simulink model "untitled"  (R2023a)
settings: Solver=VariableStepAuto  StartTime=0.0  StopTime=5.0  RelTol=1e-3
libraries: dspvision x3, dspadpt3 x2, commchan3 x1
settings Model: Creator=Admin  LastModifiedBy=Admin

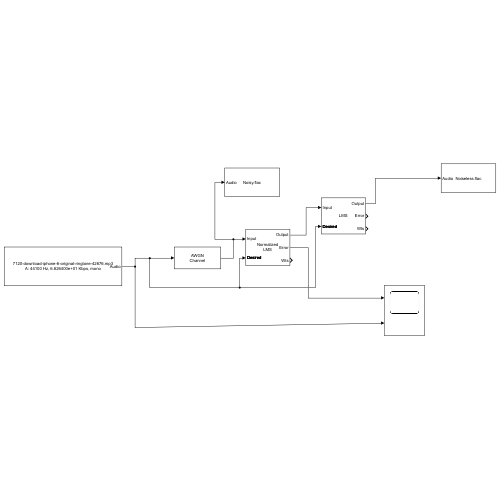
[thumbnail: Simulink's stored preview of the top-level diagram]
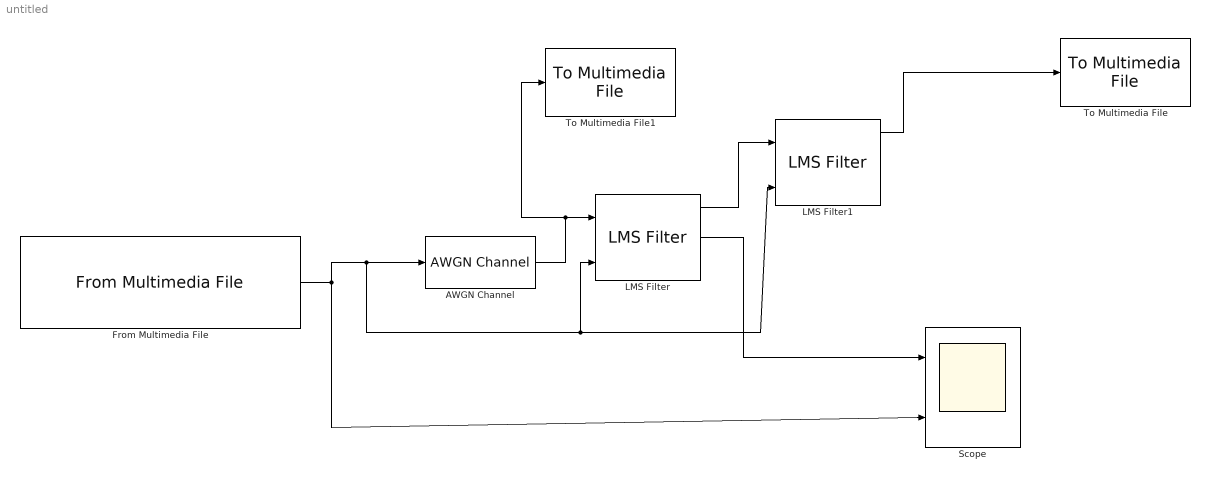
== system untitled ==
  AWGN Channel : commchan3/AWGN Channel  LegacyMode=off  NoiseMethod="Signal to noise ratio  (SNR)"  noiseMode="Signal to noise ratio  (SNR)"  EbNo=10  EsNo=10  SNR=25  BitsPerSymbol=1  SignalPower=1  SamplesPerSymbol=1  SymbolPeriod=1  VarianceSource=Parameter  Variance=1  RandomStream=Global stream  Seed=67  SimulateUsing=Code generation
  From Multimedia File : dspvision/From Multimedia File  inputFilename=C:\Users\17205\Downloads\VNIT\Folders of Courses in 8th Sem\ECP413\Project\7120-download-iphone-6-original-ringtone-42676.mp3  readRange=[1 Inf]  loop=on  numPlays=inf  outputStreams=Audio only  videoDataType=single  audioDataType=double  inheritSampleTime=on  userDefinedSampleTime=1/44100  noAudioOutput=off  isIntensityVideo=off  fourcc=RGB  colorVideoFormat=Separate color signals  outputEOF=off  dataOrg=Column-major  audioFrameSize=1024  computeAudioFrameSize=off  outSamplingMode=Sample based
      settings: LibrarySourceBlock=audiosources/From Multimedia File
  LMS Filter : dspadpt3/LMS Filter  Algo=Normalized LMS  L=100  stepflag=Dialog  mu=1  leakage=1.0  ic=0  Adapt=off  resetflag=None  weights=on  addnparflag=off  roundingMode=Floor  overflowMode=off
  LMS Filter1 : dspadpt3/LMS Filter  Algo=LMS  L=100  stepflag=Dialog  mu=0.05  leakage=1.0  ic=0  Adapt=off  resetflag=None  weights=on  addnparflag=off  roundingMode=Floor  overflowMode=off
  Scope : Scope  NumInputPorts=2
  To Multimedia File : dspvision/To Multimedia File  outputFilename=C:\Users\17205\Downloads\VNIT\Folders of Courses in 8th Sem\ECP413\Project\Noiseless.flac  streamSelection=Audio only  videoCompressor=None (uncompressed)  audioCompressor=None (uncompressed)  imagePorts=One multidimensional signal  fileType=FLAC  audioDatatype=8-bit integer  fourcc=RGB  videoQuality=75  mj2000CompFactor=10
      settings: LibrarySourceBlock=visionsinks/To Multimedia File
  To Multimedia File1 : dspvision/To Multimedia File  outputFilename=C:\Users\17205\Downloads\VNIT\Folders of Courses in 8th Sem\ECP413\Project\Noisy.flac  streamSelection=Audio only  videoCompressor=None (uncompressed)  audioCompressor=None (uncompressed)  imagePorts=One multidimensional signal  fileType=FLAC  audioDatatype=8-bit integer  fourcc=RGB  videoQuality=75  mj2000CompFactor=10
      settings: LibrarySourceBlock=visionsinks/To Multimedia File
  wires:
  From Multimedia File/1 -> LMS Filter/2, LMS Filter1/2, AWGN Channel/1, Scope/2
  AWGN Channel/1 -> To Multimedia File1/1, LMS Filter/1
  LMS Filter/2 -> Scope/1
  LMS Filter/1 -> LMS Filter1/1
  LMS Filter1/1 -> To Multimedia File/1
